simulink model "Factorial_WhileLoop"  (R2021a)
settings: Solver=VariableStepAuto  StartTime=0.0  StopTime=10.0  RelTol=1e-3
settings Model: Creator=Moamen_Hamed  LastModifiedBy=Moamen_Hamed

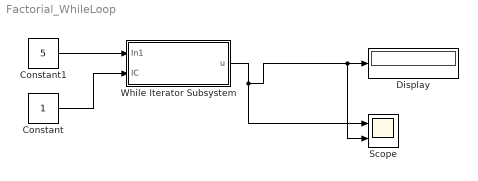
== system Factorial_WhileLoop ==
  Constant : Constant  OutDataTypeStr=int32
  Constant1 : Constant  Value=5  OutDataTypeStr=int32
  Display : Display
  Scope : Scope  NumInputPorts=2
  While Iterator Subsystem : Subsystem  TreatAsAtomicUnit=on
  wires:
  While Iterator Subsystem/1(u) -> Scope/2, Display/1, Scope/1
  Constant1/1 -> While Iterator Subsystem/1(In1)
  Constant/1 -> While Iterator Subsystem/2(IC)

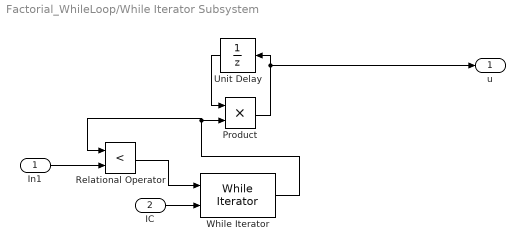
== system Factorial_WhileLoop/While Iterator Subsystem ==
  In1 : Inport
  IC : Inport  Port=2
  Product : Product  OutDataTypeStr=int32
  Relational Operator : RelationalOperator  Operator=<  OutDataTypeStr=boolean  RndMeth=Simplest
  Unit Delay : UnitDelay  InitialCondition=1  SampleTime=-1  HasFrameUpgradeWarning=on
  While Iterator : WhileIterator  MaxIters=20  ShowIterationPort=on
  u : Outport
  wires:
  IC/1 -> While Iterator/2
  Relational Operator/1 -> While Iterator/1
  In1/1 -> Relational Operator/2
  Product/1 -> u/1, Unit Delay/1
  Unit Delay/1 -> Product/1
  While Iterator/1 -> Relational Operator/1, Product/2
